simulink model "JCBL_buck_DBHR2018b"  (R2018b)
settings: Solver=VariableStepAuto  StartTime=0.0  StopTime=0.005  RelTol=1e-3
libraries: powerlib x17, simulink x2, powerlib_meascontrol x2
settings Model: Creator=admin  LastModifiedBy=admin
settings SolverCC: ZeroCrossAlgorithm=Adaptive
settings DataIOCC: ReturnWorkspaceOutputs=on

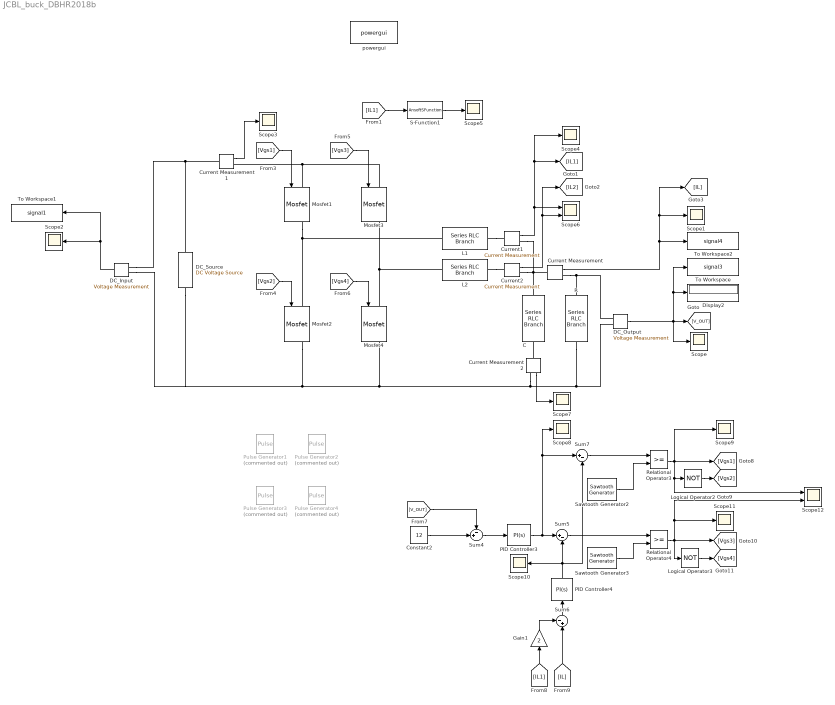
== system JCBL_buck_DBHR2018b ==
  C : powerlib/Elements/Series RLC Branch  LConnTagsString=__new0  RConnTagsString=__new0  BranchType=RC  Resistance=0.0623968564680311  Inductance=1e-3  SetiL0=off  InitialCurrent=0  Capacitance=25/3/8/2/500000/0.12  Setx0=off  InitialVoltage=0  Measurements=None
  Constant2 : Constant  Value=12
  Current Measurement : powerlib/Measurements/Current Measurement  PhasorSimulation=off  OutputType=Complex  PSBequivalent=0
  Current Measurement1 : powerlib/Measurements/Current Measurement  PhasorSimulation=off  OutputType=Complex  PSBequivalent=0
  Current Measurement2 : powerlib/Measurements/Current Measurement  PhasorSimulation=off  OutputType=Complex  PSBequivalent=0
  Current1 : powerlib/Measurements/Current Measurement  PhasorSimulation=off  OutputType=Complex  PSBequivalent=0
  Current2 : powerlib/Measurements/Current Measurement  PhasorSimulation=off  OutputType=Complex  PSBequivalent=0
  DC_Input : powerlib/Measurements/Voltage Measurement  PhasorSimulation=off  OutputType=Complex  PSBequivalent=0
  DC_Output : powerlib/Measurements/Voltage Measurement  PhasorSimulation=off  OutputType=Complex  PSBequivalent=0
  DC_Source : powerlib/Electrical Sources/DC Voltage Source  Amplitude=48  Measurements=None
  Display2 : Display
  Gain1 : Gain  Gain=2
  L1 : powerlib/Elements/Series RLC Branch  LConnTagsString=__new0  RConnTagsString=__new0  BranchType=RL  Resistance=0.1  Inductance=36*12*3/48/500000/25  SetiL0=off  InitialCurrent=0  Capacitance=1e-6  Setx0=off  InitialVoltage=0  Measurements=None
  L2 : powerlib/Elements/Series RLC Branch  LConnTagsString=__new0  RConnTagsString=__new0  BranchType=RL  Resistance=0.1  Inductance=36*12*3/48/500000/25  SetiL0=off  InitialCurrent=0  Capacitance=1e-6  Setx0=off  InitialVoltage=0  Measurements=None
  Logical Operator2 : Logic  Operator=NOT  AllPortsSameDT=off  OutDataTypeStr=boolean
  Logical Operator3 : Logic  Operator=NOT  AllPortsSameDT=off  OutDataTypeStr=boolean
  Mosfet{1..4} (4 alike) : powerlib/Power Electronics/Mosfet  Ron=0.0138704114739210  Lon=0  Rd=0.0001  Vfd=0  IC=0  Rs=1e5  Cs=inf  Measurements=on
  PID Controller3 : simulink/Continuous/PID Controller  Controller=PI  Form=Parallel  TimeDomain=Continuous-time  SampleTime=-1  IntegratorMethod=Forward Euler  FilterMethod=Forward Euler  ControllerParametersSource=internal  P=1000  I=5000  D=0  UseFilter=on  N=100  TunerSelectOption=Transfer Function Based (PID Tuner App)  InitialConditionSource=internal  InitialConditionForIntegrator=0  InitialConditionForFilter=0  DifferentiatorICPrevScaledInput=0  ExternalReset=none  TrackingMode=off  Kt=1  LimitOutput=on  UpperSaturationLimit=4  LowerSaturationLimit=-4  LinearizeAsGain=on  AntiWindupMode=none  Kb=1  POutMin=[]  POutMax=[]  IOutMin=[]  IOutMax=[]  DOutMin=[]  DOutMax=[]  NOutMin=[]  NOutMax=[]  SumOutMin=[]  SumOutMax=[]  SaturationOutMin=[]  SaturationOutMax=[]  PParamMin=[]  PParamMax=[]  IParamMin=[]  IParamMax=[]  DParamMin=[]  DParamMax=[]  NParamMin=[]  NParamMax=[]  KbParamMin=[]  KbParamMax=[]  KtParamMin=[]  KtParamMax=[]  KbOutMin=[]  KbOutMax=[]  KtOutMin=[]  KtOutMax=[]  IntegratorOutMin=[]  IntegratorOutMax=[]  FilterOutMin=[]  FilterOutMax=[]  SumI1OutMin=[]  SumI1OutMax=[]  SumI2OutMin=[]  SumI2OutMax=[]  SumI3OutMin=[]  SumI3OutMax=[]  SumI4OutMin=[]  SumI4OutMax=[]  SumDOutMin=[]  SumDOutMax=[]  DifferentiatorOutMin=[]  DifferentiatorOutMax=[]  FilterDiffOutCoefMin=[]  FilterDiffOutCoefMax=[]  ReciprocalOutMin=[]  ReciprocalOutMax=[]  SumDenOutMin=[]  SumDenOutMax=[]  SumNumOutMin=[]  SumNumOutMax=[]  DivideOutMin=[]  DivideOutMax=[]  IntegratorContinuousStateAttributes=''  IntegratorStateMustResolveToSignalObject=off  IntegratorRTWStateStorageClass=Auto  FilterContinuousStateAttributes=''  FilterStateMustResolveToSignalObject=off  FilterRTWStateStorageClass=Auto  ParallelPVariant=InternalParameters  IdealPVariant=Disabled  IVariant=InternalParameters  DVariant=Disabled  IntegratorVariant=Continuous  SatVariant=Enabled  AWVariant=Passthrough  PCopyVariant=Disabled  TRVariant=Disabled  FdbkBlocksVariant=Forward  IdealPFdbkVariant=Disabled  SatFdbkVariant=Disabled  DerivativeFilterVariant=Disabled  NVariant=Disabled  NCopyVariant=Disabled_SignalSpec  FilterICVariant=Disabled  IntegratorICVariant=InternalICs  ExternalResetVariant=Disabled  TRSumVariant=Passthrough  SumFdbkVariant=Disabled  SumVariant=Sum_PI
  PID Controller4 : simulink/Continuous/PID Controller  Controller=PI  Form=Parallel  TimeDomain=Continuous-time  SampleTime=-1  IntegratorMethod=Forward Euler  FilterMethod=Forward Euler  ControllerParametersSource=internal  P=0.05  I=1500  D=0  UseFilter=on  N=100  TunerSelectOption=Transfer Function Based (PID Tuner App)  InitialConditionSource=internal  InitialConditionForIntegrator=0  InitialConditionForFilter=0  DifferentiatorICPrevScaledInput=0  ExternalReset=none  TrackingMode=off  Kt=1  LimitOutput=on  UpperSaturationLimit=0.95  LowerSaturationLimit=-0.95  LinearizeAsGain=on  AntiWindupMode=none  Kb=1  POutMin=[]  POutMax=[]  IOutMin=[]  IOutMax=[]  DOutMin=[]  DOutMax=[]  NOutMin=[]  NOutMax=[]  SumOutMin=[]  SumOutMax=[]  SaturationOutMin=[]  SaturationOutMax=[]  PParamMin=[]  PParamMax=[]  IParamMin=[]  IParamMax=[]  DParamMin=[]  DParamMax=[]  NParamMin=[]  NParamMax=[]  KbParamMin=[]  KbParamMax=[]  KtParamMin=[]  KtParamMax=[]  KbOutMin=[]  KbOutMax=[]  KtOutMin=[]  KtOutMax=[]  IntegratorOutMin=[]  IntegratorOutMax=[]  FilterOutMin=[]  FilterOutMax=[]  SumI1OutMin=[]  SumI1OutMax=[]  SumI2OutMin=[]  SumI2OutMax=[]  SumI3OutMin=[]  SumI3OutMax=[]  SumI4OutMin=[]  SumI4OutMax=[]  SumDOutMin=[]  SumDOutMax=[]  DifferentiatorOutMin=[]  DifferentiatorOutMax=[]  FilterDiffOutCoefMin=[]  FilterDiffOutCoefMax=[]  ReciprocalOutMin=[]  ReciprocalOutMax=[]  SumDenOutMin=[]  SumDenOutMax=[]  SumNumOutMin=[]  SumNumOutMax=[]  DivideOutMin=[]  DivideOutMax=[]  IntegratorContinuousStateAttributes=''  IntegratorStateMustResolveToSignalObject=off  IntegratorRTWStateStorageClass=Auto  FilterContinuousStateAttributes=''  FilterStateMustResolveToSignalObject=off  FilterRTWStateStorageClass=Auto  ParallelPVariant=InternalParameters  IdealPVariant=Disabled  IVariant=InternalParameters  DVariant=Disabled  IntegratorVariant=Continuous  SatVariant=Enabled  AWVariant=Passthrough  PCopyVariant=Disabled  TRVariant=Disabled  FdbkBlocksVariant=Forward  IdealPFdbkVariant=Disabled  SatFdbkVariant=Disabled  DerivativeFilterVariant=Disabled  NVariant=Disabled  NCopyVariant=Disabled_SignalSpec  FilterICVariant=Disabled  IntegratorICVariant=InternalICs  ExternalResetVariant=Disabled  TRSumVariant=Passthrough  SumFdbkVariant=Disabled  SumVariant=Sum_PI
  Pulse Generator1 : DiscretePulseGenerator  Commented=on  PulseType=Time based  Period=1/461208  PulseWidth=25
  Pulse Generator2 : DiscretePulseGenerator  Commented=on  PulseType=Time based  Period=1/461208  PulseWidth=25  PhaseDelay=2/1844832
  Pulse Generator3 : DiscretePulseGenerator  Commented=on  PulseType=Time based  Period=1/461208  PulseWidth=25  PhaseDelay=1/1844832
  Pulse Generator4 : DiscretePulseGenerator  Commented=on  PulseType=Time based  Period=1/461208  PulseWidth=25  PhaseDelay=3/1844832
  R : powerlib/Elements/Series RLC Branch  LConnTagsString=__new0  RConnTagsString=__new0  BranchType=R  Resistance=0.072  Inductance=1e-3  SetiL0=off  InitialCurrent=0  Capacitance=1e-6  Setx0=off  InitialVoltage=0  Measurements=None
  Relational Operator3 : RelationalOperator  OutDataTypeStr=boolean  RndMeth=Simplest
  Relational Operator4 : RelationalOperator  OutDataTypeStr=boolean  RndMeth=Simplest
  S-Function1 : S-Function  FunctionName=AnsoftSFunction  Parameters=-1  SFunctionDeploymentMode=off  EnableBusSupport=off
      settings: OpenFcn=AnsoftLinkDialog();
  Sawtooth Generator2 : powerlib_meascontrol/Pulse & Signal Generators/Sawtooth Generator  Freq=500e3  Phase=0  Ts=0
      settings: SourceProductName=Simscape Power Systems
  Sawtooth Generator3 : powerlib_meascontrol/Pulse & Signal Generators/Sawtooth Generator  Freq=500e3  Phase=180  Ts=0
      settings: SourceProductName=Simscape Power Systems
  Scope{,1..5,7..11} (11 alike) : Scope
  Scope12 : Scope  NumInputPorts=2
  Scope6 : Scope  NumInputPorts=2
  Sum4 : Sum  Inputs=-+|
  Sum5 : Sum  Inputs=|+-
  Sum6 : Sum  Inputs=-+|
  Sum7 : Sum  Inputs=|+-
  To Workspace : ToWorkspace  VariableName=signal3  SampleTime=0.1
  To Workspace1 : ToWorkspace  VariableName=signal1  SampleTime=0.1
  To Workspace2 : ToWorkspace  VariableName=signal4  SampleTime=0.1
  powergui : powerlib/powergui  Priority=1  SimulationMode=Discrete  SampleTime=1e-7  frequency=60  Iterations=50  frequencyindice=0  Pbase=100e6  ErrMax=1e-4  UnitsV=kV  UnitsW=MW  buscounter=0  FunctionMessages=off  echomessages=off  EnableUseOfTLC=off  CurrentSourceSwitches=off  DisableSnubberDevices=off  DisableRonSwitches=off  DisableVfSwitches=off  DisplayEquations=off  SolverType=Tustin/Backward Euler (TBE)  Interpol=off  ExternalGateDelay=off  methode=off  Ts=100  x0status=blocks  SPID=on  SwTol=0  HookPort=off  RestoreLinks=warning  ResistiveCurrentMeasurement=off  Frange=[0:2:500]  Ylog=off  Xlog=on  ShowGrid=off  save=off  variable=ZData  structure=0  ZoomFFT=off  StartTime=0.0  cycles=1  DisplayStyle=1  fundamental=60  FreqAxis=off  MaxFrequency=1000  frequencyindicesteady=1  RmsSteady=1  display=off
  wires:
  DC_Output/1 -> Scope/1, Display2/1, To Workspace/1, [V_OUT]
  DC_Input/1 -> To Workspace1/1, Scope2/1
  Current Measurement/1 -> To Workspace2/1, [IL], Scope1/1
  Current Measurement1/1 -> Scope3/1
  Current1/1 -> Scope4/1, [IL1], Scope6/1
  Current2/1 -> [IL2], Scope6/2
  Constant2/1 -> Sum4/2
  [V_OUT] -> Sum4/1
  Sum4/1 -> PID Controller3/1
  PID Controller3/1 -> Scope8/1, Sum7/1, Sum5/1
  Gain1/1 -> Sum6/1
  [IL1] -> Gain1/1
  [IL] -> Sum6/2
  Sum6/1 -> PID Controller4/1
  PID Controller4/1 -> Sum5/2, Sum7/2, Scope10/1
  Sum7/1 -> Relational Operator3/1
  Sawtooth Generator2/1 -> Relational Operator3/2
  Sum5/1 -> Relational Operator4/1
  Sawtooth Generator3/1 -> Relational Operator4/2
  Logical Operator2/1 -> [Vgs2]
  Relational Operator3/1 -> Scope12/1, Logical Operator2/1, Scope9/1, [Vgs1]
  Logical Operator3/1 -> [Vgs4]
  Relational Operator4/1 -> Scope12/2, Scope11/1, Logical Operator3/1, [Vgs3]
  Current Measurement2/1 -> Scope7/1
  [Vgs1] -> Mosfet1/1
  [Vgs3] -> Mosfet3/1
  [Vgs2] -> Mosfet2/1
  [Vgs4] -> Mosfet4/1
  [IL1] -> S-Function1/1
  S-Function1/1 -> Scope5/1
  connections:
  Mosfet1/RConn1 -- Mosfet2/LConn1 -- L1/LConn1
  Mosfet1/LConn1 -- Mosfet3/LConn1 -- Current Measurement1/RConn1
  R/RConn1 -- DC_Output/LConn2 -- Current Measurement2/RConn1 -- Mosfet4/RConn1 -- DC_Source/LConn1 -- DC_Input/LConn2 -- Mosfet2/RConn1
  DC_Source/RConn1 -- DC_Input/LConn1 -- Current Measurement1/LConn1
  Mosfet4/LConn1 -- Mosfet3/RConn1 -- L2/LConn1
  C/LConn1 -- Current1/RConn1 -- Current Measurement/LConn1 -- Current2/RConn1
  Current Measurement/RConn1 -- DC_Output/LConn1 -- R/LConn1
  L2/RConn1 -- Current2/LConn1
  L1/RConn1 -- Current1/LConn1
  Current Measurement2/LConn1 -- C/RConn1
